simulink model "coupled_HBG"  (Simulink 7.5)
settings: Solver=ode4  StartTime=0.0  StopTime=3  FixedStep=0.005  MaxStep=1e-3  RelTol=1e-3
settings Model: Creator=Slim  LastModifiedBy=Slim

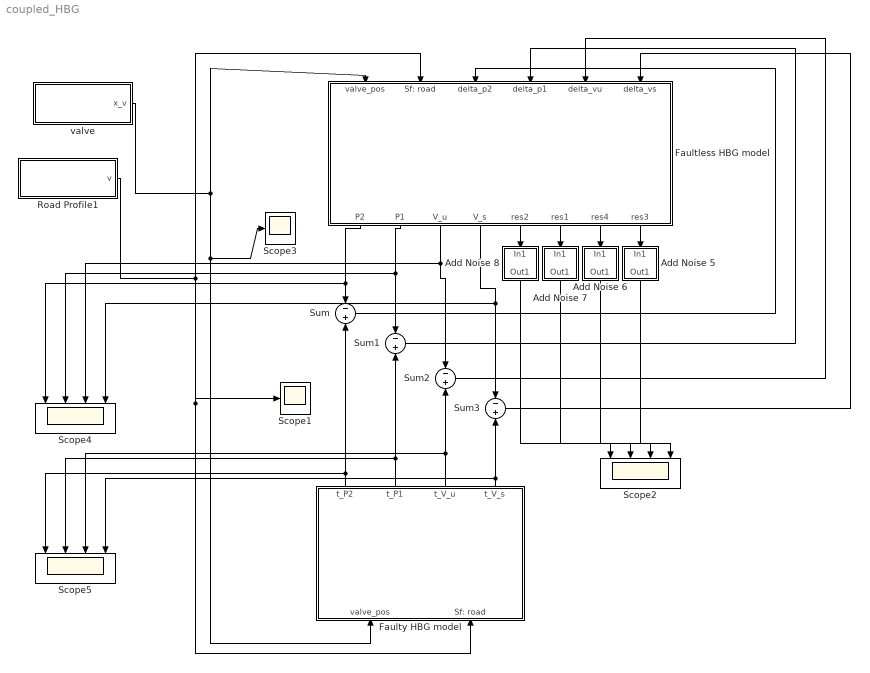
== system coupled_HBG ==
  Add Noise 5 : Subsystem  TreatAsAtomicUnit=on  mask{N=10}
      mask prompts: N "Noise"
  Add Noise 6 : Subsystem  TreatAsAtomicUnit=on  mask{N=10}
      mask prompts: N "Noise"
  Add Noise 7 : Subsystem  TreatAsAtomicUnit=on  mask{N=10}
      mask prompts: N "Noise"
  Add Noise 8 : Subsystem  TreatAsAtomicUnit=on  mask{N=10}
      mask prompts: N "Noise"
  Faultless HBG model : Subsystem
  Faulty HBG model : Subsystem
  Road Profile1 : Subsystem
  Scope1 : Scope
      settings: YMin=-1.25e+007  YMax=1.25e+007  SaveName=ScopeData2  MaxDataPoints=500000
  Scope2 : Scope  NumInputPorts=4
      settings: YMin=-4e+054~-7.5e+054~-1e+039~-1e+039  YMax=5e+054~7.5e+054~1e+040~1e+040  MaxDataPoints=500000
  Scope3 : Scope
      settings: YMin=-1.25e+007  YMax=1.25e+007  SaveName=ScopeData3  MaxDataPoints=500000
  Scope4 : Scope  NumInputPorts=4
      settings: YMin=-4e+054~-7.5e+054~-1e+039~-1e+039  YMax=5e+054~7.5e+054~1e+040~1e+040  MaxDataPoints=500000
  Scope5 : Scope  NumInputPorts=4
      settings: YMin=-4e+054~-7.5e+054~-1e+039~-1e+039  YMax=5e+054~7.5e+054~1e+040~1e+040  SaveName=ScopeData10  MaxDataPoints=500000
  Sum{,1..3} (4 alike) : Sum  Inputs=-+  OutDataType=fixdt(1, 16)  OutScaling=2^0
  valve : Subsystem
  wires:
  valve/1(x_v) -> Faultless HBG model/1(valve_pos), Faulty HBG model/1(valve_pos), Scope3/1
  Road Profile1/1(v) -> Faultless HBG model/2(Sf: road), Faulty HBG model/2(Sf: road), Scope1/1
  Faulty HBG model/1(t_P2) -> Sum/2, Scope5/1
  Faulty HBG model/2(t_P1) -> Sum1/2, Scope5/2
  Faulty HBG model/3(t_V_u) -> Sum2/2, Scope5/3
  Faulty HBG model/4(t_V_s) -> Sum3/2, Scope5/4
  Faultless HBG model/1(P2) -> Sum/1, Scope4/1
  Faultless HBG model/2(P1) -> Sum1/1, Scope4/2
  Faultless HBG model/3(V_u) -> Sum2/1, Scope4/3
  Faultless HBG model/4(V_s) -> Sum3/1, Scope4/4
  Faultless HBG model/6(res1) -> Add Noise 7/1(In1)
  Faultless HBG model/5(res2) -> Add Noise 8/1(In1)
  Faultless HBG model/8(res3) -> Add Noise 5/1(In1)
  Faultless HBG model/7(res4) -> Add Noise 6/1(In1)
  Sum/1 -> Faultless HBG model/3(delta_p2)
  Sum1/1 -> Faultless HBG model/4(delta_p1)
  Sum2/1 -> Faultless HBG model/5(delta_vu)
  Sum3/1 -> Faultless HBG model/6(delta_vs)
  Add Noise 5/1(Out1) -> Scope2/3
  Add Noise 6/1(Out1) -> Scope2/4
  Add Noise 7/1(Out1) -> Scope2/1
  Add Noise 8/1(Out1) -> Scope2/2

== system coupled_HBG/Add Noise 5 ==
  In1 : Inport
  Constant : Constant
  Gain : Gain  Gain=N/100  SaturateOnIntegerOverflow=on  OutDataTypeStr=Inherit: Same as input  ParamDataTypeStr=Inherit: Same as input
  MATLAB Fcn : MATLABFcn  MATLABFcn=randn  OutputDimensions=1
  Product : Product  SaturateOnIntegerOverflow=on  RndMeth=Zero  InputSameDT=on  OutDataTypeStr=Inherit: Same as first input
  Sum2 : Sum  Inputs=|++  SaturateOnIntegerOverflow=on  InputSameDT=on  OutDataTypeStr=Inherit: Same as first input
  Out1 : Outport  InitialOutput=0
  wires:
  Constant/1 -> MATLAB Fcn/1
  Gain/1 -> Product/2
  Product/1 -> Sum2/2
  MATLAB Fcn/1 -> Gain/1
  In1/1 -> Product/1, Sum2/1
  Sum2/1 -> Out1/1

== system coupled_HBG/Add Noise 6 ==
  In1 : Inport
  Constant : Constant
  Gain : Gain  Gain=N/100  SaturateOnIntegerOverflow=on  OutDataTypeStr=Inherit: Same as input  ParamDataTypeStr=Inherit: Same as input
  MATLAB Fcn : MATLABFcn  MATLABFcn=randn  OutputDimensions=1
  Product : Product  SaturateOnIntegerOverflow=on  RndMeth=Zero  InputSameDT=on  OutDataTypeStr=Inherit: Same as first input
  Sum2 : Sum  Inputs=|++  SaturateOnIntegerOverflow=on  InputSameDT=on  OutDataTypeStr=Inherit: Same as first input
  Out1 : Outport  InitialOutput=0
  wires:
  Sum2/1 -> Out1/1
  In1/1 -> Sum2/1, Product/1
  MATLAB Fcn/1 -> Gain/1
  Product/1 -> Sum2/2
  Gain/1 -> Product/2
  Constant/1 -> MATLAB Fcn/1

== system coupled_HBG/Add Noise 7 ==
  In1 : Inport
  Constant : Constant
  Gain : Gain  Gain=N/100  SaturateOnIntegerOverflow=on  OutDataTypeStr=Inherit: Same as input  ParamDataTypeStr=Inherit: Same as input
  MATLAB Fcn : MATLABFcn  MATLABFcn=randn  OutputDimensions=1
  Product : Product  SaturateOnIntegerOverflow=on  RndMeth=Zero  InputSameDT=on  OutDataTypeStr=Inherit: Same as first input
  Sum2 : Sum  Inputs=|++  SaturateOnIntegerOverflow=on  InputSameDT=on  OutDataTypeStr=Inherit: Same as first input
  Out1 : Outport  InitialOutput=0
  wires:
  Constant/1 -> MATLAB Fcn/1
  Gain/1 -> Product/2
  Product/1 -> Sum2/2
  MATLAB Fcn/1 -> Gain/1
  In1/1 -> Product/1, Sum2/1
  Sum2/1 -> Out1/1

== system coupled_HBG/Add Noise 8 ==
  In1 : Inport
  Constant : Constant
  Gain : Gain  Gain=N/100  SaturateOnIntegerOverflow=on  OutDataTypeStr=Inherit: Same as input  ParamDataTypeStr=Inherit: Same as input
  MATLAB Fcn : MATLABFcn  MATLABFcn=randn  OutputDimensions=1
  Product : Product  SaturateOnIntegerOverflow=on  RndMeth=Zero  InputSameDT=on  OutDataTypeStr=Inherit: Same as first input
  Sum2 : Sum  Inputs=|++  SaturateOnIntegerOverflow=on  InputSameDT=on  OutDataTypeStr=Inherit: Same as first input
  Out1 : Outport  InitialOutput=0
  wires:
  Sum2/1 -> Out1/1
  In1/1 -> Sum2/1, Product/1
  MATLAB Fcn/1 -> Gain/1
  Product/1 -> Sum2/2
  Gain/1 -> Product/2
  Constant/1 -> MATLAB Fcn/1

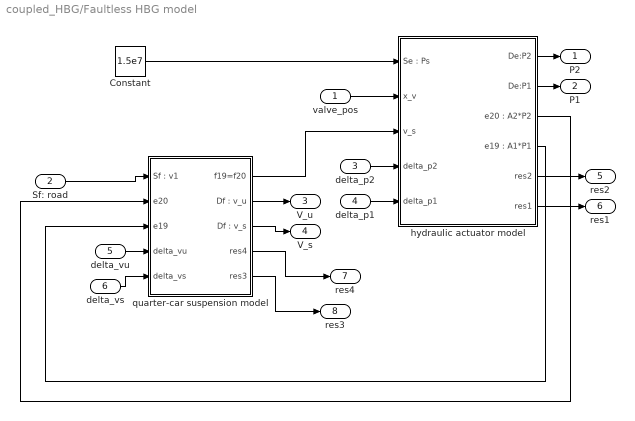
== system coupled_HBG/Faultless HBG model ==
  valve_pos : Inport
  Sf: road : Inport  Port=2
  delta_p2 : Inport  Port=3
  delta_p1 : Inport  Port=4
  delta_vu : Inport  Port=5
  delta_vs : Inport  Port=6
  Constant : Constant  Value=1.5e7  OutDataType=fixdt(1, 16)  OutScaling=2^0
  hydraulic actuator model : Subsystem
  quarter-car suspension model : Subsystem
  P2 : Outport
  P1 : Outport  Port=2
  V_u : Outport  Port=3
  V_s : Outport  Port=4
  res2 : Outport  Port=5
  res1 : Outport  Port=6
  res4 : Outport  Port=7
  res3 : Outport  Port=8
  wires:
  quarter-car suspension model/1(f19=f20) -> hydraulic actuator model/3(v_s)
  hydraulic actuator model/1(De:P2) -> P2/1
  Constant/1 -> hydraulic actuator model/1("Se : Ps")
  hydraulic actuator model/2(De:P1) -> P1/1
  valve_pos/1 -> hydraulic actuator model/2(x_v)
  hydraulic actuator model/3("e20 : A2*P2") -> quarter-car suspension model/2(e20)
  Sf: road/1 -> quarter-car suspension model/1("Sf : v1")
  hydraulic actuator model/4("e19 : A1*P1") -> quarter-car suspension model/3(e19)
  quarter-car suspension model/2("Df : v_u") -> V_u/1
  quarter-car suspension model/3("Df : v_s") -> V_s/1
  delta_p2/1 -> hydraulic actuator model/4(delta_p2)
  delta_p1/1 -> hydraulic actuator model/5(delta_p1)
  delta_vs/1 -> quarter-car suspension model/5(delta_vs)
  delta_vu/1 -> quarter-car suspension model/4(delta_vu)
  hydraulic actuator model/5(res2) -> res2/1
  hydraulic actuator model/6(res1) -> res1/1
  quarter-car suspension model/4(res4) -> res4/1
  quarter-car suspension model/5(res3) -> res3/1

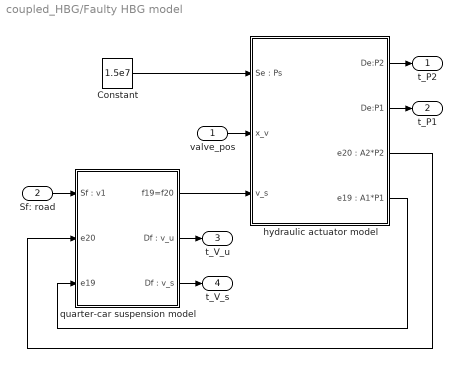
== system coupled_HBG/Faulty HBG model ==
  valve_pos : Inport
  Sf: road : Inport  Port=2
  Constant : Constant  Value=1.5e7  OutDataType=fixdt(1, 16)  OutScaling=2^0
  hydraulic actuator model : Subsystem
  quarter-car suspension model : Subsystem
  t_P2 : Outport
  t_P1 : Outport  Port=2
  t_V_u : Outport  Port=3
  t_V_s : Outport  Port=4
  wires:
  quarter-car suspension model/3("Df : v_s") -> t_V_s/1
  quarter-car suspension model/2("Df : v_u") -> t_V_u/1
  hydraulic actuator model/4("e19 : A1*P1") -> quarter-car suspension model/3(e19)
  Sf: road/1 -> quarter-car suspension model/1("Sf : v1")
  hydraulic actuator model/3("e20 : A2*P2") -> quarter-car suspension model/2(e20)
  valve_pos/1 -> hydraulic actuator model/2(x_v)
  hydraulic actuator model/2(De:P1) -> t_P1/1
  Constant/1 -> hydraulic actuator model/1("Se : Ps")
  hydraulic actuator model/1(De:P2) -> t_P2/1
  quarter-car suspension model/1(f19=f20) -> hydraulic actuator model/3(v_s)

== system coupled_HBG/Road Profile1 ==
  Clock : Clock
      settings: Decimation=10
  Constant : Constant  Value=0.05  OutDataType=fixdt(1, 16)  OutScaling=2^0
  Derivative : Derivative
  Fcn : Fcn  Expr=0.05/2-0.05/2*cos(2*pi*12.5/5*u(1))
  Switch : Switch  Criteria=u2 > Threshold  Threshold=5/12.5*0.5  OutDataType=fixdt(1, 16)  OutScaling=2^0
  v : Outport  OutDataType=fixdt(1, 16)  OutScaling=2^0
  wires:
  Derivative/1 -> v/1
  Switch/1 -> Derivative/1
  Fcn/1 -> Switch/3
  Constant/1 -> Switch/1
  Clock/1 -> Switch/2, Fcn/1

== system coupled_HBG/valve ==
  Mux1 : Mux  Inputs=2
  Scope1 : Scope
      settings: YMin=6.25e-037  YMax=8.75e-037  SaveName=ScopeData7
  Sine Wave : Sin  Amplitude=2  Bias=0  Frequency=pi  Phase=0  Samples=10  SampleTime=0  Offset=0
  Transfer Fcn : TransferFcn  Denominator=[1/314^2 2*0.7/314 1]
  x_v : Outport  OutDataType=fixdt(1, 16)  OutScaling=2^0
  wires:
  Mux1/1 -> Scope1/1
  Sine Wave/1 -> Mux1/1, Transfer Fcn/1
  Transfer Fcn/1 -> Mux1/2, x_v/1

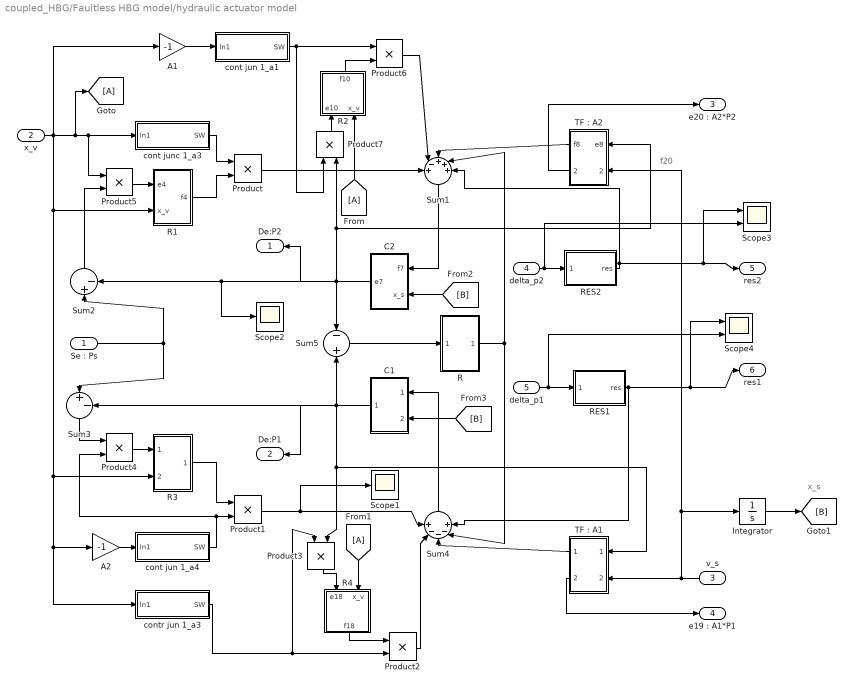
== system coupled_HBG/Faultless HBG model/hydraulic actuator model ==
  note: x_s
  note: f20
  "Se : Ps" : Inport  OutDataType=fixdt(1, 16)  OutScaling=2^0
  x_v : Inport  Port=2  OutDataType=fixdt(1, 16)  OutScaling=2^0
  v_s : Inport  Port=3  OutDataType=fixdt(1, 16)  OutScaling=2^0
  delta_p2 : Inport  Port=4  OutDataType=fixdt(1, 16)  OutScaling=2^0
  delta_p1 : Inport  Port=5  OutDataType=fixdt(1, 16)  OutScaling=2^0
  A1 : Gain  Gain=-1  ParameterDataType=fixdt(1, 16)  ParameterScaling=2^0  OutDataType=fixdt(1, 16)  OutScaling=2^0
  A2 : Gain  Gain=-1  ParameterDataType=fixdt(1, 16)  ParameterScaling=2^0  OutDataType=fixdt(1, 16)  OutScaling=2^0
  C1 : Subsystem
  C2 : Subsystem
  Integrator : Integrator
  Product{,1..7} (8 alike) : Product  OutDataType=fixdt(1, 16)  OutScaling=2^0  RndMeth=Zero
  R : Subsystem
  R1 : Subsystem
  R2 : Subsystem
  R3 : Subsystem
  R4 : Subsystem
  RES1 : Subsystem
  RES2 : Subsystem
  Scope1 : Scope
      settings: YMin=-1.25e+007  YMax=1.25e+007  SaveName=ScopeData6
  Scope2 : Scope
      settings: YMin=-1.25e+007  YMax=1.25e+007  SaveName=ScopeData5
  Scope3 : Scope  NumInputPorts=2
      settings: YMin=-1.25e+007~-5  YMax=1.25e+007~5  SaveName=ScopeData4
  Scope4 : Scope  NumInputPorts=2
      settings: YMin=-1.25e+007~-5  YMax=1.25e+007~5  SaveName=ScopeData8
  Sum1 : Sum  Inputs=+-+++  OutDataType=fixdt(1, 16)  OutScaling=2^0
  Sum2 : Sum  Inputs=|+-  OutDataType=fixdt(1, 16)  OutScaling=2^0
  Sum3 : Sum  Inputs=|+-  OutDataType=fixdt(1, 16)  OutScaling=2^0
  Sum4 : Sum  Inputs=+---+  OutDataType=fixdt(1, 16)  OutScaling=2^0
  Sum5 : Sum  Inputs=-+  OutDataType=fixdt(1, 16)  OutScaling=2^0
  "TF : A1" : Subsystem
  "TF : A2" : Subsystem
  cont jun 1_a1 : Subsystem
  cont jun 1_a4 : Subsystem
  cont junc 1_a3 : Subsystem
  contr jun 1_a3 : Subsystem
  De:P2 : Outport  OutDataType=fixdt(1, 16)  OutScaling=2^0
  De:P1 : Outport  Port=2  OutDataType=fixdt(1, 16)  OutScaling=2^0
  "e20 : A2*P2" : Outport  Port=3  OutDataType=fixdt(1, 16)  OutScaling=2^0
  "e19 : A1*P1" : Outport  Port=4  OutDataType=fixdt(1, 16)  OutScaling=2^0
  res2 : Outport  Port=5  OutDataType=fixdt(1, 16)  OutScaling=2^0
  res1 : Outport  Port=6  OutDataType=fixdt(1, 16)  OutScaling=2^0
  wires:
  Product7/1 -> R2/1(e10)
  Product6/1 -> Sum1/2
  R2/1(f10) -> Product6/2
  cont jun 1_a1/1(SW) -> Product7/1, Product6/1
  A1/1 -> cont jun 1_a1/1(In1)
  Product5/1 -> R1/1(e4)
  Product4/1 -> R3/1(e14)
  Product3/1 -> R4/1(e18)
  Product2/1 -> Sum4/2
  R4/1(f18) -> Product2/1
  contr jun 1_a3/1(SW) -> Product3/1, Product2/2
  Sum3/1 -> Product4/1
  Sum2/1 -> Product5/2
  [B] -> C1/2(x_s)
  [B] -> C2/2(x_s)
  Integrator/1 -> [B]
  [A] -> R4/2(x_v)
  [A] -> R2/2(x_v)
  A2/1 -> cont jun 1_a4/1(In1)
  x_v/1 -> A1/1, R1/2(x_v), contr jun 1_a3/1(In1), A2/1, R3/2(x_v), Product5/1, cont junc 1_a3/1(In1), [A]
  "TF : A2"/2(e20) -> "e20 : A2*P2"/1
  "TF : A1"/2(e19) -> "e19 : A1*P1"/1
  v_s/1 -> Integrator/1, "TF : A2"/2(f20), "TF : A1"/2(f19)
  "TF : A1"/1(f17) -> Sum4/3
  "TF : A2"/1(f8) -> Sum1/3
  R/1(f11) -> Sum4/4, Sum1/4
  Product1/1 -> Scope1/1, Sum4/1
  Sum5/1 -> R/1(e11)
  Sum4/1 -> C1/1(f16)
  C1/1(e16) -> Product3/2, "TF : A1"/1(e17), De:P1/1, Sum5/2, Sum3/2
  Product/1 -> Sum1/1
  R3/1(f14) -> Product1/1
  cont jun 1_a4/1(SW) -> Product4/2, Product1/2
  Sum1/1 -> C2/1(f7)
  C2/1(e7) -> Product7/2, "TF : A2"/1(e8), De:P2/1, Sum5/1, Sum2/2, Scope2/1
  R1/1(f4) -> Product/2
  cont junc 1_a3/1(SW) -> Product/1
  "Se : Ps"/1 -> Sum3/1, Sum2/1
  delta_p2/1 -> RES2/1(delta_e), Scope3/2
  RES2/1(res) -> Sum1/5, res2/1, Scope3/1
  delta_p1/1 -> RES1/1(delta_e), Scope4/2
  RES1/1(res) -> Sum4/5, res1/1, Scope4/1

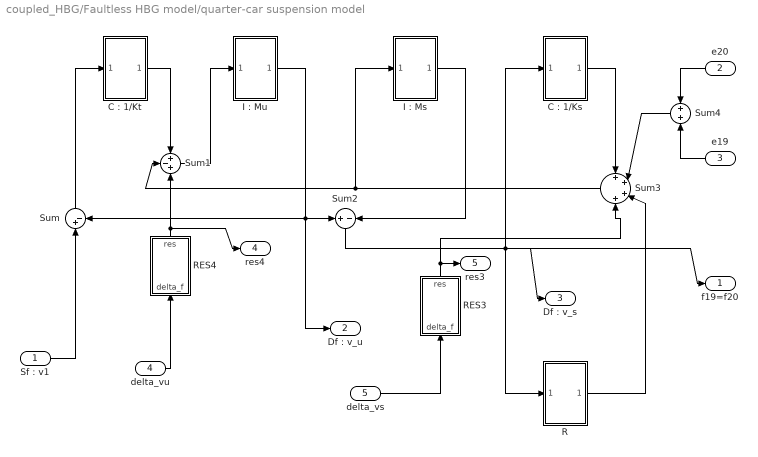
== system coupled_HBG/Faultless HBG model/quarter-car suspension model ==
  "Sf : v1" : Inport  OutDataType=fixdt(1, 16)  OutScaling=2^0
  e20 : Inport  Port=2  OutDataType=fixdt(1, 16)  OutScaling=2^0
  e19 : Inport  Port=3  OutDataType=fixdt(1, 16)  OutScaling=2^0
  delta_vu : Inport  Port=4  OutDataType=fixdt(1, 16)  OutScaling=2^0
  delta_vs : Inport  Port=5  OutDataType=fixdt(1, 16)  OutScaling=2^0
  "C : 1/Ks" : Subsystem
  "C : 1/Kt" : Subsystem
  "I : Ms" : Subsystem
  "I : Mu" : Subsystem
  R : Subsystem
  RES3 : Subsystem
  RES4 : Subsystem
  Sum : Sum  Inputs=|+-  OutDataType=fixdt(1, 16)  OutScaling=2^0
  Sum1 : Sum  Inputs=+-+  OutDataType=fixdt(1, 16)  OutScaling=2^0
  Sum2 : Sum  Inputs=+-  OutDataType=fixdt(1, 16)  OutScaling=2^0
  Sum3 : Sum  Inputs=++++  OutDataType=fixdt(1, 16)  OutScaling=2^0
  Sum4 : Sum  OutDataType=fixdt(1, 16)  OutScaling=2^0
  f19=f20 : Outport  OutDataType=fixdt(1, 16)  OutScaling=2^0
  "Df : v_u" : Outport  Port=2  OutDataType=fixdt(1, 16)  OutScaling=2^0
  "Df : v_s" : Outport  Port=3  OutDataType=fixdt(1, 16)  OutScaling=2^0
  res4 : Outport  Port=4  OutDataType=fixdt(1, 16)  OutScaling=2^0
  res3 : Outport  Port=5  OutDataType=fixdt(1, 16)  OutScaling=2^0
  wires:
  R/1(e23) -> Sum3/3
  "C : 1/Ks"/1(e21) -> Sum3/1
  Sum2/1 -> "Df : v_s"/1, f19=f20/1, R/1(f23), "C : 1/Ks"/1(f21)
  Sum3/1 -> "I : Ms"/1(e24), Sum1/2
  "I : Ms"/1(f24) -> Sum2/2
  "I : Mu"/1(f26) -> "Df : v_u"/1, Sum/2, Sum2/1
  Sum1/1 -> "I : Mu"/1(e26)
  "C : 1/Kt"/1(e28) -> Sum1/1
  Sum/1 -> "C : 1/Kt"/1(f28)
  "Sf : v1"/1 -> Sum/1
  delta_vu/1 -> RES4/1(delta_f)
  RES4/1(res) -> Sum1/3, res4/1
  delta_vs/1 -> RES3/1(delta_f)
  RES3/1(res) -> res3/1, Sum3/4
  e20/1 -> Sum4/1
  e19/1 -> Sum4/2
  Sum4/1 -> Sum3/2

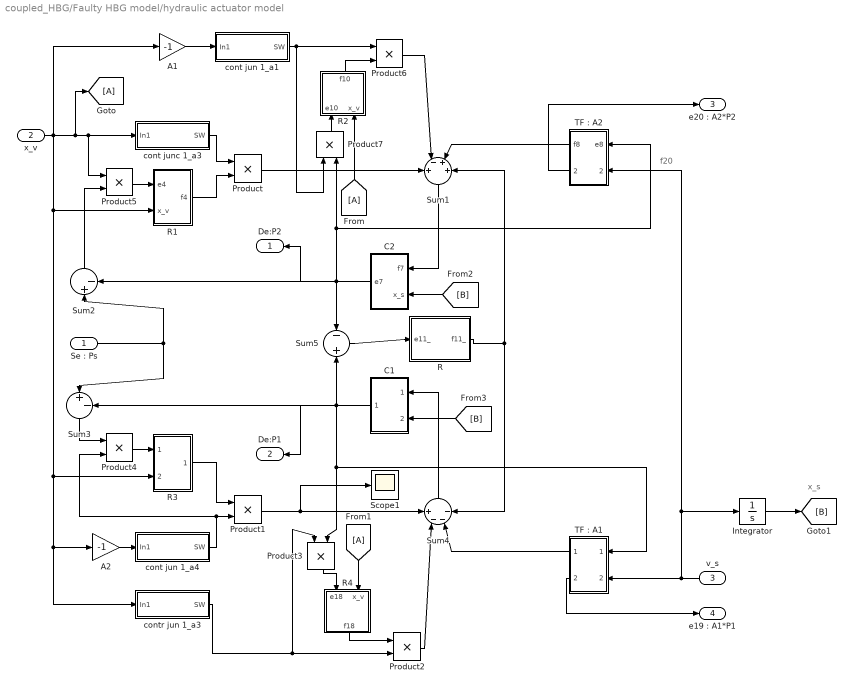
== system coupled_HBG/Faulty HBG model/hydraulic actuator model ==
  note: f20
  note: x_s
  "Se : Ps" : Inport  OutDataType=fixdt(1, 16)  OutScaling=2^0
  x_v : Inport  Port=2  OutDataType=fixdt(1, 16)  OutScaling=2^0
  v_s : Inport  Port=3  OutDataType=fixdt(1, 16)  OutScaling=2^0
  A1 : Gain  Gain=-1  ParameterDataType=fixdt(1, 16)  ParameterScaling=2^0  OutDataType=fixdt(1, 16)  OutScaling=2^0
  A2 : Gain  Gain=-1  ParameterDataType=fixdt(1, 16)  ParameterScaling=2^0  OutDataType=fixdt(1, 16)  OutScaling=2^0
  C1 : Subsystem
  C2 : Subsystem
  Integrator : Integrator
  Product{,1..7} (8 alike) : Product  OutDataType=fixdt(1, 16)  OutScaling=2^0  RndMeth=Zero
  R : Subsystem  TreatAsAtomicUnit=on  mask{R=0.3e-12, FM=0.4, FT=1.2, FTe=1.8}
      mask prompts: R "Resistance"; FM "Fault Magnitude"; FT "Fault Time Start"; FTe "Fault Time End"
  R1 : Subsystem
  R2 : Subsystem
  R3 : Subsystem
  R4 : Subsystem
  Scope1 : Scope
      settings: YMin=-1.25e+007  YMax=1.25e+007  SaveName=ScopeData6
  Sum1 : Sum  Inputs=+-++  OutDataType=fixdt(1, 16)  OutScaling=2^0
  Sum2 : Sum  Inputs=|+-  OutDataType=fixdt(1, 16)  OutScaling=2^0
  Sum3 : Sum  Inputs=|+-  OutDataType=fixdt(1, 16)  OutScaling=2^0
  Sum4 : Sum  Inputs=+---  OutDataType=fixdt(1, 16)  OutScaling=2^0
  Sum5 : Sum  Inputs=-+  OutDataType=fixdt(1, 16)  OutScaling=2^0
  "TF : A1" : Subsystem
  "TF : A2" : Subsystem
  cont jun 1_a1 : Subsystem
  cont jun 1_a4 : Subsystem
  cont junc 1_a3 : Subsystem
  contr jun 1_a3 : Subsystem
  De:P2 : Outport  OutDataType=fixdt(1, 16)  OutScaling=2^0
  De:P1 : Outport  Port=2  OutDataType=fixdt(1, 16)  OutScaling=2^0
  "e20 : A2*P2" : Outport  Port=3  OutDataType=fixdt(1, 16)  OutScaling=2^0
  "e19 : A1*P1" : Outport  Port=4  OutDataType=fixdt(1, 16)  OutScaling=2^0
  wires:
  "Se : Ps"/1 -> Sum2/1, Sum3/1
  cont junc 1_a3/1(SW) -> Product/1
  R1/1(f4) -> Product/2
  C2/1(e7) -> Sum2/2, Sum5/1, De:P2/1, "TF : A2"/1(e8), Product7/2
  Sum1/1 -> C2/1(f7)
  cont jun 1_a4/1(SW) -> Product1/2, Product4/2
  R3/1(f14) -> Product1/1
  Product/1 -> Sum1/1
  C1/1(e16) -> Sum3/2, Sum5/2, De:P1/1, "TF : A1"/1(e17), Product3/2
  Sum4/1 -> C1/1(f16)
  Sum5/1 -> R/1(e11_)
  Product1/1 -> Sum4/1, Scope1/1
  R/1(f11_) -> Sum1/4, Sum4/4
  "TF : A2"/1(f8) -> Sum1/3
  "TF : A1"/1(f17) -> Sum4/3
  v_s/1 -> "TF : A1"/2(f19), "TF : A2"/2(f20), Integrator/1
  "TF : A1"/2(e19) -> "e19 : A1*P1"/1
  "TF : A2"/2(e20) -> "e20 : A2*P2"/1
  x_v/1 -> [A], cont junc 1_a3/1(In1), Product5/1, R3/2(x_v), A2/1, contr jun 1_a3/1(In1), R1/2(x_v), A1/1
  A2/1 -> cont jun 1_a4/1(In1)
  [A] -> R2/2(x_v)
  [A] -> R4/2(x_v)
  Integrator/1 -> [B]
  [B] -> C2/2(x_s)
  [B] -> C1/2(x_s)
  Sum2/1 -> Product5/2
  Sum3/1 -> Product4/1
  contr jun 1_a3/1(SW) -> Product2/2, Product3/1
  R4/1(f18) -> Product2/1
  Product2/1 -> Sum4/2
  Product3/1 -> R4/1(e18)
  Product4/1 -> R3/1(e14)
  Product5/1 -> R1/1(e4)
  A1/1 -> cont jun 1_a1/1(In1)
  cont jun 1_a1/1(SW) -> Product6/1, Product7/1
  R2/1(f10) -> Product6/2
  Product6/1 -> Sum1/2
  Product7/1 -> R2/1(e10)

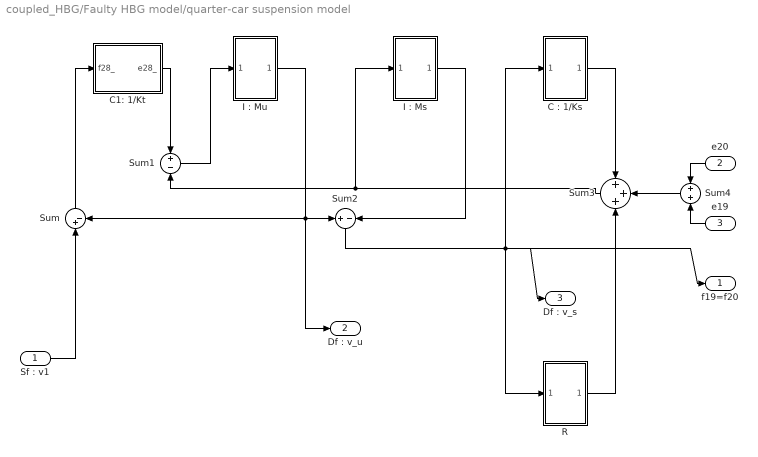
== system coupled_HBG/Faulty HBG model/quarter-car suspension model ==
  "Sf : v1" : Inport  OutDataType=fixdt(1, 16)  OutScaling=2^0
  e20 : Inport  Port=2  OutDataType=fixdt(1, 16)  OutScaling=2^0
  e19 : Inport  Port=3  OutDataType=fixdt(1, 16)  OutScaling=2^0
  "C : 1/Ks" : Subsystem
  C1: 1/Kt : Subsystem  TreatAsAtomicUnit=on  mask{C=1/190000, FM=1, FT=0, FTe=0}
      mask prompts: C "Capacitance"; FM "Fault Magnitude"; FT "Fault Time Start"; FTe "Fault Time End"
  "I : Ms" : Subsystem
  "I : Mu" : Subsystem
  R : Subsystem
  Sum : Sum  Inputs=|+-  OutDataType=fixdt(1, 16)  OutScaling=2^0
  Sum1 : Sum  Inputs=+-  OutDataType=fixdt(1, 16)  OutScaling=2^0
  Sum2 : Sum  Inputs=+-  OutDataType=fixdt(1, 16)  OutScaling=2^0
  Sum3 : Sum  Inputs=+++  OutDataType=fixdt(1, 16)  OutScaling=2^0
  Sum4 : Sum  OutDataType=fixdt(1, 16)  OutScaling=2^0
  f19=f20 : Outport  OutDataType=fixdt(1, 16)  OutScaling=2^0
  "Df : v_u" : Outport  Port=2  OutDataType=fixdt(1, 16)  OutScaling=2^0
  "Df : v_s" : Outport  Port=3  OutDataType=fixdt(1, 16)  OutScaling=2^0
  wires:
  "Sf : v1"/1 -> Sum/1
  C1: 1/Kt/1(e28_) -> Sum1/1
  Sum1/1 -> "I : Mu"/1(e26)
  "I : Mu"/1(f26) -> Sum2/1, Sum/2, "Df : v_u"/1
  "I : Ms"/1(f24) -> Sum2/2
  Sum3/1 -> Sum1/2, "I : Ms"/1(e24)
  Sum2/1 -> "C : 1/Ks"/1(f21), R/1(f23), f19=f20/1, "Df : v_s"/1
  "C : 1/Ks"/1(e21) -> Sum3/1
  R/1(e23) -> Sum3/3
  Sum/1 -> C1: 1/Kt/1(f28_)
  e20/1 -> Sum4/1
  e19/1 -> Sum4/2
  Sum4/1 -> Sum3/2

== system coupled_HBG/Faultless HBG model/hydraulic actuator model/C1 ==
  f16 : Inport  OutDataType=fixdt(1, 16)  OutScaling=2^0
  x_s : Inport  Port=2  OutDataType=fixdt(1, 16)  OutScaling=2^0
  Fcn : Fcn  Expr=1.2e9/(1.2e-4-3.8e-4*u(1))
  Integrator : Integrator
  Product : Product  OutDataType=fixdt(1, 16)  OutScaling=2^0  RndMeth=Zero
  e16 : Outport  OutDataType=fixdt(1, 16)  OutScaling=2^0
  wires:
  Product/1 -> e16/1
  Fcn/1 -> Product/2
  x_s/1 -> Fcn/1
  Integrator/1 -> Product/1
  f16/1 -> Integrator/1

== system coupled_HBG/Faultless HBG model/hydraulic actuator model/C2 ==
  f7 : Inport  OutDataType=fixdt(1, 16)  OutScaling=2^0
  x_s : Inport  Port=2  OutDataType=fixdt(1, 16)  OutScaling=2^0
  Fcn : Fcn  Expr=1.2e9/(1.1e-4+3.5e-4*u(1))
  Integrator : Integrator
  Product : Product  OutDataType=fixdt(1, 16)  OutScaling=2^0  RndMeth=Zero
  e7 : Outport  OutDataType=fixdt(1, 16)  OutScaling=2^0
  wires:
  Product/1 -> e7/1
  Fcn/1 -> Product/2
  Integrator/1 -> Product/1
  f7/1 -> Integrator/1
  x_s/1 -> Fcn/1

== system coupled_HBG/Faultless HBG model/hydraulic actuator model/R ==
  e11 : Inport  OutDataType=fixdt(1, 16)  OutScaling=2^0
  1/Ctm : Gain  Gain=0.3e-12  ParameterDataType=fixdt(1, 16)  ParameterScaling=2^0  OutDataType=fixdt(1, 16)  OutScaling=2^0
  f11 : Outport  OutDataType=fixdt(1, 16)  OutScaling=2^0
  wires:
  1/Ctm/1 -> f11/1
  e11/1 -> 1/Ctm/1

== system coupled_HBG/Faultless HBG model/hydraulic actuator model/R1 ==
  e4 : Inport  OutDataType=fixdt(1, 16)  OutScaling=2^0
  x_v : Inport  Port=2  OutDataType=fixdt(1, 16)  OutScaling=2^0
  Fcn : Fcn  Expr=-0.6*1.5e-3*u(2)*sqrt(2/900*abs(u(1)))
  Mux : Mux  Inputs=2
  f4 : Outport  OutDataType=fixdt(1, 16)  OutScaling=2^0
  wires:
  Fcn/1 -> f4/1
  Mux/1 -> Fcn/1
  e4/1 -> Mux/1
  x_v/1 -> Mux/2

== system coupled_HBG/Faultless HBG model/hydraulic actuator model/R2 ==
  e10 : Inport  OutDataType=fixdt(1, 16)  OutScaling=2^0
  x_v : Inport  Port=2  OutDataType=fixdt(1, 16)  OutScaling=2^0
  Fcn : Fcn  Expr=0.6*1.5e-3*u(2)*sqrt(2/900*abs(u(1)))
  Mux : Mux  Inputs=2
  f10 : Outport  OutDataType=fixdt(1, 16)  OutScaling=2^0
  wires:
  Fcn/1 -> f10/1
  Mux/1 -> Fcn/1
  x_v/1 -> Mux/2
  e10/1 -> Mux/1

== system coupled_HBG/Faultless HBG model/hydraulic actuator model/R3 ==
  e14 : Inport  OutDataType=fixdt(1, 16)  OutScaling=2^0
  x_v : Inport  Port=2  OutDataType=fixdt(1, 16)  OutScaling=2^0
  Fcn : Fcn  Expr=-0.6*1.5e-3*u(2)*sqrt(2/900*abs(u(1)))
  Mux : Mux  Inputs=2
  f14 : Outport  OutDataType=fixdt(1, 16)  OutScaling=2^0
  wires:
  x_v/1 -> Mux/2
  e14/1 -> Mux/1
  Fcn/1 -> f14/1
  Mux/1 -> Fcn/1

== system coupled_HBG/Faultless HBG model/hydraulic actuator model/R4 ==
  e18 : Inport  OutDataType=fixdt(1, 16)  OutScaling=2^0
  x_v : Inport  Port=2  OutDataType=fixdt(1, 16)  OutScaling=2^0
  Fcn : Fcn  Expr=0.6*1.5e-3*u(2)*sqrt(2/900*abs(u(1)))
  Mux : Mux  Inputs=2
  f18 : Outport  OutDataType=fixdt(1, 16)  OutScaling=2^0
  wires:
  x_v/1 -> Mux/2
  e18/1 -> Mux/1
  Mux/1 -> Fcn/1
  Fcn/1 -> f18/1

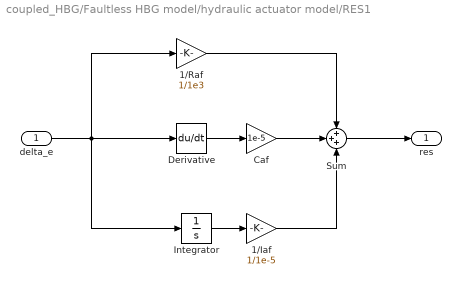
== system coupled_HBG/Faultless HBG model/hydraulic actuator model/RES1 ==
  delta_e : Inport  OutDataType=fixdt(1, 16)  OutScaling=2^0
  1/Iaf : Gain  Gain=1/1e-5  ParameterDataType=fixdt(1, 16)  ParameterScaling=2^0  OutDataType=fixdt(1, 16)  OutScaling=2^0
  1/Raf : Gain  Gain=1/1e3  ParameterDataType=fixdt(1, 16)  ParameterScaling=2^0  OutDataType=fixdt(1, 16)  OutScaling=2^0
  Caf : Gain  Gain=1e-5  ParameterDataType=fixdt(1, 16)  ParameterScaling=2^0  OutDataType=fixdt(1, 16)  OutScaling=2^0
  Derivative : Derivative
  Integrator : Integrator
  Sum : Sum  Inputs=+++  OutDataType=fixdt(1, 16)  OutScaling=2^0
  res : Outport  OutDataType=fixdt(1, 16)  OutScaling=2^0
  wires:
  Sum/1 -> res/1
  1/Iaf/1 -> Sum/3
  Caf/1 -> Sum/2
  1/Raf/1 -> Sum/1
  Derivative/1 -> Caf/1
  Integrator/1 -> 1/Iaf/1
  delta_e/1 -> Integrator/1, Derivative/1, 1/Raf/1

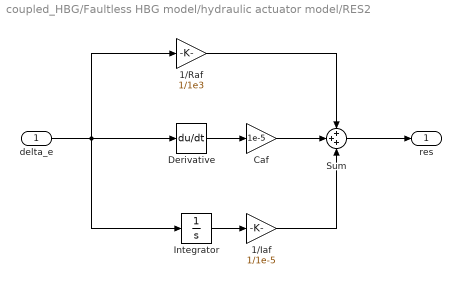
== system coupled_HBG/Faultless HBG model/hydraulic actuator model/RES2 ==
  delta_e : Inport  OutDataType=fixdt(1, 16)  OutScaling=2^0
  1/Iaf : Gain  Gain=1/1e-5  ParameterDataType=fixdt(1, 16)  ParameterScaling=2^0  OutDataType=fixdt(1, 16)  OutScaling=2^0
  1/Raf : Gain  Gain=1/1e3  ParameterDataType=fixdt(1, 16)  ParameterScaling=2^0  OutDataType=fixdt(1, 16)  OutScaling=2^0
  Caf : Gain  Gain=1e-5  ParameterDataType=fixdt(1, 16)  ParameterScaling=2^0  OutDataType=fixdt(1, 16)  OutScaling=2^0
  Derivative : Derivative
  Integrator : Integrator
  Sum : Sum  Inputs=+++  OutDataType=fixdt(1, 16)  OutScaling=2^0
  res : Outport  OutDataType=fixdt(1, 16)  OutScaling=2^0
  wires:
  delta_e/1 -> 1/Raf/1, Derivative/1, Integrator/1
  Integrator/1 -> 1/Iaf/1
  Derivative/1 -> Caf/1
  1/Raf/1 -> Sum/1
  Caf/1 -> Sum/2
  1/Iaf/1 -> Sum/3
  Sum/1 -> res/1

== system coupled_HBG/Faultless HBG model/hydraulic actuator model/TF : A1 ==
  e17 : Inport  OutDataType=fixdt(1, 16)  OutScaling=2^0
  f19 : Inport  Port=2  OutDataType=fixdt(1, 16)  OutScaling=2^0
  A2 : Gain  Gain=3.8e-4  ParameterDataType=fixdt(1, 16)  ParameterScaling=2^0  OutDataType=fixdt(1, 16)  OutScaling=2^0
  "TF : A1" : Gain  Gain=3.8e-4  ParameterDataType=fixdt(1, 16)  ParameterScaling=2^0  OutDataType=fixdt(1, 16)  OutScaling=2^0
  f17 : Outport  OutDataType=fixdt(1, 16)  OutScaling=2^0
  e19 : Outport  Port=2  OutDataType=fixdt(1, 16)  OutScaling=2^0
  wires:
  f19/1 -> "TF : A1"/1
  "TF : A1"/1 -> f17/1
  e17/1 -> A2/1
  A2/1 -> e19/1

== system coupled_HBG/Faultless HBG model/hydraulic actuator model/TF : A2 ==
  e8 : Inport  OutDataType=fixdt(1, 16)  OutScaling=2^0
  f20 : Inport  Port=2  OutDataType=fixdt(1, 16)  OutScaling=2^0
  A2 : Gain  Gain=3.5e-4  ParameterDataType=fixdt(1, 16)  ParameterScaling=2^0  OutDataType=fixdt(1, 16)  OutScaling=2^0
  "TF : A2" : Gain  Gain=3.5e-4  ParameterDataType=fixdt(1, 16)  ParameterScaling=2^0  OutDataType=fixdt(1, 16)  OutScaling=2^0
  f8 : Outport  OutDataType=fixdt(1, 16)  OutScaling=2^0
  e20 : Outport  Port=2  OutDataType=fixdt(1, 16)  OutScaling=2^0
  wires:
  A2/1 -> e20/1
  e8/1 -> A2/1
  "TF : A2"/1 -> f8/1
  f20/1 -> "TF : A2"/1

== system coupled_HBG/Faultless HBG model/hydraulic actuator model/cont jun 1_a1 ==
  In1 : Inport  OutDataType=fixdt(1, 16)  OutScaling=2^0
  Constant : Constant  OutDataType=sfix(16)  OutScaling=2^0
  Constant1 : Constant  Value=0  OutDataType=sfix(16)  OutScaling=2^0
  Switch : Switch  Criteria=u2 > Threshold  OutDataType=sfix(16)  OutScaling=2^0
  SW : Outport  OutDataType=fixdt(1, 16)  OutScaling=2^0
  wires:
  In1/1 -> Switch/2
  Constant1/1 -> Switch/3
  Constant/1 -> Switch/1
  Switch/1 -> SW/1

== system coupled_HBG/Faultless HBG model/hydraulic actuator model/cont jun 1_a4 ==
  In1 : Inport  OutDataType=fixdt(1, 16)  OutScaling=2^0
  Constant : Constant  OutDataType=sfix(16)  OutScaling=2^0
  Constant1 : Constant  Value=0  OutDataType=sfix(16)  OutScaling=2^0
  Switch : Switch  Criteria=u2 > Threshold  OutDataType=sfix(16)  OutScaling=2^0
  SW : Outport  OutDataType=fixdt(1, 16)  OutScaling=2^0
  wires:
  Switch/1 -> SW/1
  Constant/1 -> Switch/1
  Constant1/1 -> Switch/3
  In1/1 -> Switch/2

== system coupled_HBG/Faultless HBG model/hydraulic actuator model/cont junc 1_a3 ==
  In1 : Inport  OutDataType=fixdt(1, 16)  OutScaling=2^0
  Constant : Constant  OutDataType=sfix(16)  OutScaling=2^0
  Constant1 : Constant  Value=0  OutDataType=sfix(16)  OutScaling=2^0
  Switch : Switch  OutDataType=sfix(16)  OutScaling=2^0
  SW : Outport  OutDataType=fixdt(1, 16)  OutScaling=2^0
  wires:
  In1/1 -> Switch/2
  Constant1/1 -> Switch/3
  Constant/1 -> Switch/1
  Switch/1 -> SW/1

== system coupled_HBG/Faultless HBG model/hydraulic actuator model/contr jun 1_a3 ==
  In1 : Inport  OutDataType=fixdt(1, 16)  OutScaling=2^0
  Constant : Constant  OutDataType=sfix(16)  OutScaling=2^0
  Constant1 : Constant  Value=0  OutDataType=sfix(16)  OutScaling=2^0
  Switch : Switch  OutDataType=sfix(16)  OutScaling=2^0
  SW : Outport  OutDataType=fixdt(1, 16)  OutScaling=2^0
  wires:
  Switch/1 -> SW/1
  Constant/1 -> Switch/1
  Constant1/1 -> Switch/3
  In1/1 -> Switch/2

== system coupled_HBG/Faultless HBG model/quarter-car suspension model/C : 1/Ks ==
  f21 : Inport  OutDataType=fixdt(1, 16)  OutScaling=2^0
  1/C1 : Gain  Gain=16800  ParameterDataType=fixdt(1, 16)  ParameterScaling=2^0  OutDataType=fixdt(1, 16)  OutScaling=2^0
  Integrator : Integrator
  e21 : Outport  OutDataType=fixdt(1, 16)  OutScaling=2^0
  wires:
  f21/1 -> Integrator/1
  Integrator/1 -> 1/C1/1
  1/C1/1 -> e21/1

== system coupled_HBG/Faultless HBG model/quarter-car suspension model/C : 1/Kt ==
  f28 : Inport  OutDataType=fixdt(1, 16)  OutScaling=2^0
  1/C1 : Gain  Gain=190000  ParameterDataType=fixdt(1, 16)  ParameterScaling=2^0  OutDataType=fixdt(1, 16)  OutScaling=2^0
  Integrator : Integrator
  e28 : Outport  OutDataType=fixdt(1, 16)  OutScaling=2^0
  wires:
  1/C1/1 -> e28/1
  Integrator/1 -> 1/C1/1
  f28/1 -> Integrator/1

== system coupled_HBG/Faultless HBG model/quarter-car suspension model/I : Ms ==
  e24 : Inport  OutDataType=fixdt(1, 16)  OutScaling=2^0
  1/I : Gain  Gain=1/290  ParameterDataType=fixdt(1, 16)  ParameterScaling=2^0  OutDataType=fixdt(1, 16)  OutScaling=2^0
  Integrator : Integrator
  f24 : Outport  OutDataType=fixdt(1, 16)  OutScaling=2^0
  wires:
  e24/1 -> Integrator/1
  Integrator/1 -> 1/I/1
  1/I/1 -> f24/1

== system coupled_HBG/Faultless HBG model/quarter-car suspension model/I : Mu ==
  e26 : Inport  OutDataType=fixdt(1, 16)  OutScaling=2^0
  1/I : Gain  Gain=1/59  ParameterDataType=fixdt(1, 16)  ParameterScaling=2^0  OutDataType=fixdt(1, 16)  OutScaling=2^0
  Integrator : Integrator
  f26 : Outport  OutDataType=fixdt(1, 16)  OutScaling=2^0
  wires:
  1/I/1 -> f26/1
  Integrator/1 -> 1/I/1
  e26/1 -> Integrator/1

== system coupled_HBG/Faultless HBG model/quarter-car suspension model/R ==
  f23 : Inport  OutDataType=fixdt(1, 16)  OutScaling=2^0
  R : Gain  Gain=1000  ParameterDataType=fixdt(1, 16)  ParameterScaling=2^0  OutDataType=fixdt(1, 16)  OutScaling=2^0
  e23 : Outport  OutDataType=fixdt(1, 16)  OutScaling=2^0
  wires:
  f23/1 -> R/1
  R/1 -> e23/1

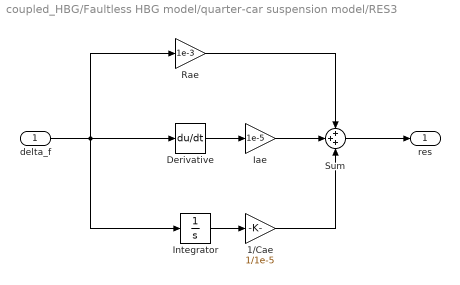
== system coupled_HBG/Faultless HBG model/quarter-car suspension model/RES3 ==
  delta_f : Inport  OutDataType=fixdt(1, 16)  OutScaling=2^0
  1/Cae : Gain  Gain=1/1e-5  ParameterDataType=fixdt(1, 16)  ParameterScaling=2^0  OutDataType=fixdt(1, 16)  OutScaling=2^0
  Derivative : Derivative
  Iae : Gain  Gain=1e-5  ParameterDataType=fixdt(1, 16)  ParameterScaling=2^0  OutDataType=fixdt(1, 16)  OutScaling=2^0
  Integrator : Integrator
  Rae : Gain  Gain=1e-3  ParameterDataType=fixdt(1, 16)  ParameterScaling=2^0  OutDataType=fixdt(1, 16)  OutScaling=2^0
  Sum : Sum  Inputs=+++  OutDataType=fixdt(1, 16)  OutScaling=2^0
  res : Outport  OutDataType=fixdt(1, 16)  OutScaling=2^0
  wires:
  delta_f/1 -> Rae/1, Derivative/1, Integrator/1
  Integrator/1 -> 1/Cae/1
  Derivative/1 -> Iae/1
  Rae/1 -> Sum/1
  Iae/1 -> Sum/2
  1/Cae/1 -> Sum/3
  Sum/1 -> res/1

== system coupled_HBG/Faultless HBG model/quarter-car suspension model/RES4 ==
  delta_f : Inport  OutDataType=fixdt(1, 16)  OutScaling=2^0
  1/Cae : Gain  Gain=1/1e-5  ParameterDataType=fixdt(1, 16)  ParameterScaling=2^0  OutDataType=fixdt(1, 16)  OutScaling=2^0
  Derivative : Derivative
  Iae : Gain  Gain=1e-5  ParameterDataType=fixdt(1, 16)  ParameterScaling=2^0  OutDataType=fixdt(1, 16)  OutScaling=2^0
  Integrator : Integrator
  Rae : Gain  Gain=1e-3  ParameterDataType=fixdt(1, 16)  ParameterScaling=2^0  OutDataType=fixdt(1, 16)  OutScaling=2^0
  Sum : Sum  Inputs=+++  OutDataType=fixdt(1, 16)  OutScaling=2^0
  res : Outport  OutDataType=fixdt(1, 16)  OutScaling=2^0
  wires:
  Sum/1 -> res/1
  1/Cae/1 -> Sum/3
  Iae/1 -> Sum/2
  Rae/1 -> Sum/1
  Derivative/1 -> Iae/1
  Integrator/1 -> 1/Cae/1
  delta_f/1 -> Integrator/1, Derivative/1, Rae/1

== system coupled_HBG/Faulty HBG model/hydraulic actuator model/C1 ==
  f16 : Inport  OutDataType=fixdt(1, 16)  OutScaling=2^0
  x_s : Inport  Port=2  OutDataType=fixdt(1, 16)  OutScaling=2^0
  Fcn : Fcn  Expr=1.2e9/(1.2e-4-3.8e-4*u(1))
  Integrator : Integrator
  Product : Product  OutDataType=fixdt(1, 16)  OutScaling=2^0  RndMeth=Zero
  e16 : Outport  OutDataType=fixdt(1, 16)  OutScaling=2^0
  wires:
  f16/1 -> Integrator/1
  Integrator/1 -> Product/1
  x_s/1 -> Fcn/1
  Fcn/1 -> Product/2
  Product/1 -> e16/1

== system coupled_HBG/Faulty HBG model/hydraulic actuator model/C2 ==
  f7 : Inport  OutDataType=fixdt(1, 16)  OutScaling=2^0
  x_s : Inport  Port=2  OutDataType=fixdt(1, 16)  OutScaling=2^0
  Fcn : Fcn  Expr=1.2e9/(1.1e-4+3.5e-4*u(1))
  Integrator : Integrator
  Product : Product  OutDataType=fixdt(1, 16)  OutScaling=2^0  RndMeth=Zero
  e7 : Outport  OutDataType=fixdt(1, 16)  OutScaling=2^0
  wires:
  x_s/1 -> Fcn/1
  f7/1 -> Integrator/1
  Integrator/1 -> Product/1
  Fcn/1 -> Product/2
  Product/1 -> e7/1

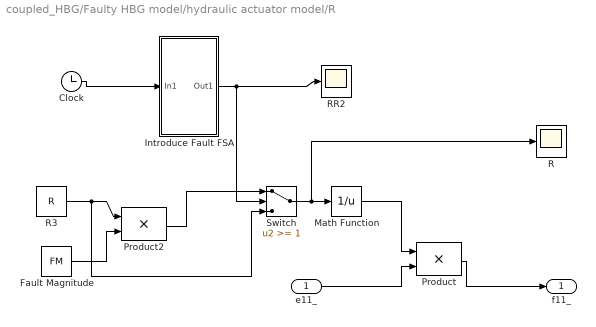
== system coupled_HBG/Faulty HBG model/hydraulic actuator model/R ==
  e11_ : Inport
  Clock : Clock
      settings: Decimation=10
  Fault Magnitude : Constant  Value=FM
  Introduce Fault FSA : Subsystem
  Math Function : Math  Operator=reciprocal  SaturateOnIntegerOverflow=on
  Product : Product  SaturateOnIntegerOverflow=on  RndMeth=Zero  InputSameDT=on  OutDataTypeStr=Inherit: Same as first input
  Product2 : Product  SaturateOnIntegerOverflow=on  RndMeth=Zero  InputSameDT=on  OutDataTypeStr=Inherit: Same as first input
  R : Scope
      settings: YMin=0  YMax=0.6  MaxDataPoints=500000
  R3 : Constant  Value=R
  RR2 : Scope
      settings: YMin=0  YMax=0.6  SaveName=ScopeData15  MaxDataPoints=500000
  Switch : Switch  Threshold=1  SaturateOnIntegerOverflow=on  InputSameDT=on
  f11_ : Outport  InitialOutput=0
  wires:
  Product/1 -> f11_/1
  e11_/1 -> Product/2
  Math Function/1 -> Product/1
  Clock/1 -> Introduce Fault FSA/1(In1)
  Fault Magnitude/1 -> Product2/2
  R3/1 -> Product2/1, Switch/3
  Product2/1 -> Switch/1
  Switch/1 -> Math Function/1, R/1
  Introduce Fault FSA/1(Out1) -> Switch/2, RR2/1

== system coupled_HBG/Faulty HBG model/hydraulic actuator model/R1 ==
  e4 : Inport  OutDataType=fixdt(1, 16)  OutScaling=2^0
  x_v : Inport  Port=2  OutDataType=fixdt(1, 16)  OutScaling=2^0
  Fcn : Fcn  Expr=-0.6*1.5e-3*u(2)*sqrt(2/900*abs(u(1)))
  Mux : Mux  Inputs=2
  f4 : Outport  OutDataType=fixdt(1, 16)  OutScaling=2^0
  wires:
  x_v/1 -> Mux/2
  e4/1 -> Mux/1
  Mux/1 -> Fcn/1
  Fcn/1 -> f4/1

== system coupled_HBG/Faulty HBG model/hydraulic actuator model/R2 ==
  e10 : Inport  OutDataType=fixdt(1, 16)  OutScaling=2^0
  x_v : Inport  Port=2  OutDataType=fixdt(1, 16)  OutScaling=2^0
  Fcn : Fcn  Expr=0.6*1.5e-3*u(2)*sqrt(2/900*abs(u(1)))
  Mux : Mux  Inputs=2
  f10 : Outport  OutDataType=fixdt(1, 16)  OutScaling=2^0
  wires:
  e10/1 -> Mux/1
  x_v/1 -> Mux/2
  Mux/1 -> Fcn/1
  Fcn/1 -> f10/1

== system coupled_HBG/Faulty HBG model/hydraulic actuator model/R3 ==
  e14 : Inport  OutDataType=fixdt(1, 16)  OutScaling=2^0
  x_v : Inport  Port=2  OutDataType=fixdt(1, 16)  OutScaling=2^0
  Fcn : Fcn  Expr=-0.6*1.5e-3*u(2)*sqrt(2/900*abs(u(1)))
  Mux : Mux  Inputs=2
  f14 : Outport  OutDataType=fixdt(1, 16)  OutScaling=2^0
  wires:
  Mux/1 -> Fcn/1
  Fcn/1 -> f14/1
  e14/1 -> Mux/1
  x_v/1 -> Mux/2

== system coupled_HBG/Faulty HBG model/hydraulic actuator model/R4 ==
  e18 : Inport  OutDataType=fixdt(1, 16)  OutScaling=2^0
  x_v : Inport  Port=2  OutDataType=fixdt(1, 16)  OutScaling=2^0
  Fcn : Fcn  Expr=0.6*1.5e-3*u(2)*sqrt(2/900*abs(u(1)))
  Mux : Mux  Inputs=2
  f18 : Outport  OutDataType=fixdt(1, 16)  OutScaling=2^0
  wires:
  Fcn/1 -> f18/1
  Mux/1 -> Fcn/1
  e18/1 -> Mux/1
  x_v/1 -> Mux/2

== system coupled_HBG/Faulty HBG model/hydraulic actuator model/TF : A1 ==
  e17 : Inport  OutDataType=fixdt(1, 16)  OutScaling=2^0
  f19 : Inport  Port=2  OutDataType=fixdt(1, 16)  OutScaling=2^0
  A2 : Gain  Gain=3.8e-4  ParameterDataType=fixdt(1, 16)  ParameterScaling=2^0  OutDataType=fixdt(1, 16)  OutScaling=2^0
  "TF : A1" : Gain  Gain=3.8e-4  ParameterDataType=fixdt(1, 16)  ParameterScaling=2^0  OutDataType=fixdt(1, 16)  OutScaling=2^0
  f17 : Outport  OutDataType=fixdt(1, 16)  OutScaling=2^0
  e19 : Outport  Port=2  OutDataType=fixdt(1, 16)  OutScaling=2^0
  wires:
  A2/1 -> e19/1
  e17/1 -> A2/1
  "TF : A1"/1 -> f17/1
  f19/1 -> "TF : A1"/1

== system coupled_HBG/Faulty HBG model/hydraulic actuator model/TF : A2 ==
  e8 : Inport  OutDataType=fixdt(1, 16)  OutScaling=2^0
  f20 : Inport  Port=2  OutDataType=fixdt(1, 16)  OutScaling=2^0
  A2 : Gain  Gain=3.5e-4  ParameterDataType=fixdt(1, 16)  ParameterScaling=2^0  OutDataType=fixdt(1, 16)  OutScaling=2^0
  "TF : A2" : Gain  Gain=3.5e-4  ParameterDataType=fixdt(1, 16)  ParameterScaling=2^0  OutDataType=fixdt(1, 16)  OutScaling=2^0
  f8 : Outport  OutDataType=fixdt(1, 16)  OutScaling=2^0
  e20 : Outport  Port=2  OutDataType=fixdt(1, 16)  OutScaling=2^0
  wires:
  f20/1 -> "TF : A2"/1
  "TF : A2"/1 -> f8/1
  e8/1 -> A2/1
  A2/1 -> e20/1

== system coupled_HBG/Faulty HBG model/hydraulic actuator model/cont jun 1_a1 ==
  In1 : Inport  OutDataType=fixdt(1, 16)  OutScaling=2^0
  Constant : Constant  OutDataType=sfix(16)  OutScaling=2^0
  Constant1 : Constant  Value=0  OutDataType=sfix(16)  OutScaling=2^0
  Switch : Switch  Criteria=u2 > Threshold  OutDataType=sfix(16)  OutScaling=2^0
  SW : Outport  OutDataType=fixdt(1, 16)  OutScaling=2^0
  wires:
  Switch/1 -> SW/1
  Constant/1 -> Switch/1
  Constant1/1 -> Switch/3
  In1/1 -> Switch/2

== system coupled_HBG/Faulty HBG model/hydraulic actuator model/cont jun 1_a4 ==
  In1 : Inport  OutDataType=fixdt(1, 16)  OutScaling=2^0
  Constant : Constant  OutDataType=sfix(16)  OutScaling=2^0
  Constant1 : Constant  Value=0  OutDataType=sfix(16)  OutScaling=2^0
  Switch : Switch  Criteria=u2 > Threshold  OutDataType=sfix(16)  OutScaling=2^0
  SW : Outport  OutDataType=fixdt(1, 16)  OutScaling=2^0
  wires:
  In1/1 -> Switch/2
  Constant1/1 -> Switch/3
  Constant/1 -> Switch/1
  Switch/1 -> SW/1

== system coupled_HBG/Faulty HBG model/hydraulic actuator model/cont junc 1_a3 ==
  In1 : Inport  OutDataType=fixdt(1, 16)  OutScaling=2^0
  Constant : Constant  OutDataType=sfix(16)  OutScaling=2^0
  Constant1 : Constant  Value=0  OutDataType=sfix(16)  OutScaling=2^0
  Switch : Switch  OutDataType=sfix(16)  OutScaling=2^0
  SW : Outport  OutDataType=fixdt(1, 16)  OutScaling=2^0
  wires:
  Switch/1 -> SW/1
  Constant/1 -> Switch/1
  Constant1/1 -> Switch/3
  In1/1 -> Switch/2

== system coupled_HBG/Faulty HBG model/hydraulic actuator model/contr jun 1_a3 ==
  In1 : Inport  OutDataType=fixdt(1, 16)  OutScaling=2^0
  Constant : Constant  OutDataType=sfix(16)  OutScaling=2^0
  Constant1 : Constant  Value=0  OutDataType=sfix(16)  OutScaling=2^0
  Switch : Switch  OutDataType=sfix(16)  OutScaling=2^0
  SW : Outport  OutDataType=fixdt(1, 16)  OutScaling=2^0
  wires:
  In1/1 -> Switch/2
  Constant1/1 -> Switch/3
  Constant/1 -> Switch/1
  Switch/1 -> SW/1

== system coupled_HBG/Faulty HBG model/quarter-car suspension model/C : 1/Ks ==
  f21 : Inport  OutDataType=fixdt(1, 16)  OutScaling=2^0
  1/C1 : Gain  Gain=16800  ParameterDataType=fixdt(1, 16)  ParameterScaling=2^0  OutDataType=fixdt(1, 16)  OutScaling=2^0
  Integrator : Integrator
  e21 : Outport  OutDataType=fixdt(1, 16)  OutScaling=2^0
  wires:
  1/C1/1 -> e21/1
  Integrator/1 -> 1/C1/1
  f21/1 -> Integrator/1

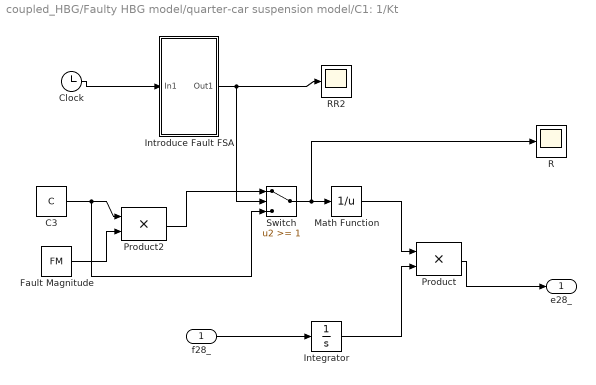
== system coupled_HBG/Faulty HBG model/quarter-car suspension model/C1: 1/Kt ==
  f28_ : Inport
  C3 : Constant  Value=C
  Clock : Clock
      settings: Decimation=10
  Fault Magnitude : Constant  Value=FM
  Integrator : Integrator
  Introduce Fault FSA : Subsystem
  Math Function : Math  Operator=reciprocal  SaturateOnIntegerOverflow=on
  Product : Product  SaturateOnIntegerOverflow=on  RndMeth=Zero  InputSameDT=on  OutDataTypeStr=Inherit: Same as first input
  Product2 : Product  SaturateOnIntegerOverflow=on  RndMeth=Zero  InputSameDT=on  OutDataTypeStr=Inherit: Same as first input
  R : Scope
      settings: YMin=0  YMax=0.6  MaxDataPoints=500000
  RR2 : Scope
      settings: YMin=0  YMax=0.6  SaveName=ScopeData15  MaxDataPoints=500000
  Switch : Switch  Threshold=1  SaturateOnIntegerOverflow=on  InputSameDT=on
  e28_ : Outport  InitialOutput=0
  wires:
  Product/1 -> e28_/1
  f28_/1 -> Integrator/1
  Math Function/1 -> Product/1
  Clock/1 -> Introduce Fault FSA/1(In1)
  Fault Magnitude/1 -> Product2/2
  C3/1 -> Product2/1, Switch/3
  Product2/1 -> Switch/1
  Switch/1 -> Math Function/1, R/1
  Introduce Fault FSA/1(Out1) -> Switch/2, RR2/1
  Integrator/1 -> Product/2

== system coupled_HBG/Faulty HBG model/quarter-car suspension model/I : Ms ==
  e24 : Inport  OutDataType=fixdt(1, 16)  OutScaling=2^0
  1/I : Gain  Gain=1/290  ParameterDataType=fixdt(1, 16)  ParameterScaling=2^0  OutDataType=fixdt(1, 16)  OutScaling=2^0
  Integrator : Integrator
  f24 : Outport  OutDataType=fixdt(1, 16)  OutScaling=2^0
  wires:
  1/I/1 -> f24/1
  Integrator/1 -> 1/I/1
  e24/1 -> Integrator/1

== system coupled_HBG/Faulty HBG model/quarter-car suspension model/I : Mu ==
  e26 : Inport  OutDataType=fixdt(1, 16)  OutScaling=2^0
  1/I : Gain  Gain=1/59  ParameterDataType=fixdt(1, 16)  ParameterScaling=2^0  OutDataType=fixdt(1, 16)  OutScaling=2^0
  Integrator : Integrator
  f26 : Outport  OutDataType=fixdt(1, 16)  OutScaling=2^0
  wires:
  e26/1 -> Integrator/1
  Integrator/1 -> 1/I/1
  1/I/1 -> f26/1

== system coupled_HBG/Faulty HBG model/quarter-car suspension model/R ==
  f23 : Inport  OutDataType=fixdt(1, 16)  OutScaling=2^0
  R : Gain  Gain=1000  ParameterDataType=fixdt(1, 16)  ParameterScaling=2^0  OutDataType=fixdt(1, 16)  OutScaling=2^0
  e23 : Outport  OutDataType=fixdt(1, 16)  OutScaling=2^0
  wires:
  R/1 -> e23/1
  f23/1 -> R/1

== system coupled_HBG/Faulty HBG model/hydraulic actuator model/R/Introduce Fault FSA ==
  In1 : Inport
  Fault Time : Constant  Value=FT
  Fault Time1 : Constant  Value=FTe
  Product : Product  OutDataType=fixdt(1, 16)  OutScaling=2^0  RndMeth=Zero
  on1 : RelationalOperator  InputSameDT=on
  on2 : RelationalOperator  Operator=<=  InputSameDT=on
  Out1 : Outport
  wires:
  Fault Time/1 -> on1/2
  In1/1 -> on1/1, on2/1
  Fault Time1/1 -> on2/2
  on1/1 -> Product/1
  on2/1 -> Product/2
  Product/1 -> Out1/1

== system coupled_HBG/Faulty HBG model/quarter-car suspension model/C1: 1/Kt/Introduce Fault FSA ==
  In1 : Inport
  Fault Time : Constant  Value=FT
  Fault Time1 : Constant  Value=FTe
  Product : Product  OutDataType=fixdt(1, 16)  OutScaling=2^0  RndMeth=Zero
  on1 : RelationalOperator  InputSameDT=on
  on2 : RelationalOperator  Operator=<=  InputSameDT=on
  Out1 : Outport
  wires:
  Fault Time/1 -> on1/2
  In1/1 -> on1/1, on2/1
  Fault Time1/1 -> on2/2
  on1/1 -> Product/1
  on2/1 -> Product/2
  Product/1 -> Out1/1
